simulink model "GOSH1"  (Simulink 8.1)
settings: Solver=ode45  StartTime=0.0  StopTime=10.0  RelTol=1e-3
libraries: simulink x1
settings Model: Creator=Mihail  LastModifiedBy=Mihail
settings DebuggingCC: FcnCallInpInsideContextMsg=EnableAllAsWarning
settings GRTTargetCC: CombineOutputUpdateFcns=on  GRTInterface=off

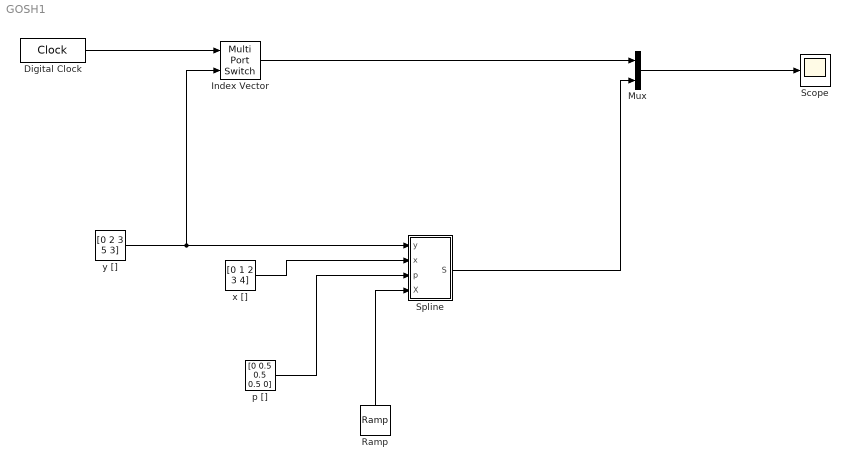
== system GOSH1 ==
  Digital Clock : DigitalClock
  Index Vector : MultiPortSwitch  DataPortOrder=Zero-based contiguous  Inputs=1  zeroidx=on
  Mux : Mux  Inputs=2
  Ramp : simulink/Sources/Ramp  slope=1  start=0  X0=0
  Scope : Scope
      settings: TimeRange=0.06668296375670701  YMin=2.961430172622083  YMax=3.275129869258235
  Spline : Subsystem
  p [] : Constant  Value=[0 0.5 0.5 0.5 0]
  x [] : Constant  Value=[0 1 2 3 4]
  y [] : Constant  Value=[0 2 3 5 3]
  wires:
  y []/1 -> Index Vector/2, Spline/1(y)
  Index Vector/1 -> Mux/1
  Digital Clock/1 -> Index Vector/1
  Mux/1 -> Scope/1
  x []/1 -> Spline/2(x)
  Ramp/1 -> Spline/4(X)
  Spline/1(S) -> Mux/2
  p []/1 -> Spline/3(p)

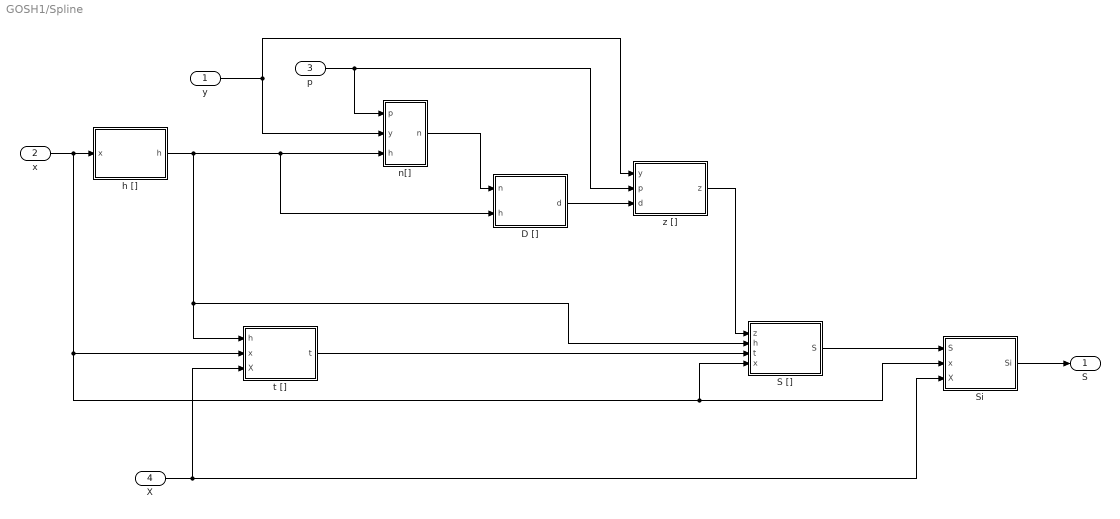
== system GOSH1/Spline ==
  y : Inport
  x : Inport  Port=2
  p : Inport  Port=3
  X : Inport  Port=4
  D [] : MATLAB Function  TreatAsAtomicUnit=on
  S [] : MATLAB Function  TreatAsAtomicUnit=on
  Si : MATLAB Function  TreatAsAtomicUnit=on
  h [] : MATLAB Function  TreatAsAtomicUnit=on
  n[] : Subsystem
  t [] : MATLAB Function  TreatAsAtomicUnit=on
  z [] : MATLAB Function  TreatAsAtomicUnit=on
  S : Outport
  wires:
  Si/1(Si) -> S/1
  S []/1(S) -> Si/1(S)
  y/1 -> n[]/2(y), z []/1(y)
  n[]/1(n) -> D []/1(n)
  X/1 -> Si/3(X), t []/3(X)
  p/1 -> n[]/1(p), z []/2(p)
  x/1 -> Si/2(x), S []/4(x), t []/2(x), h []/1(x)
  z []/1(z) -> S []/1(z)
  t []/1(t) -> S []/3(t)
  D []/1(d) -> z []/3(d)
  h []/1(h) -> t []/1(h), S []/2(h), D []/2(h), n[]/3(h)

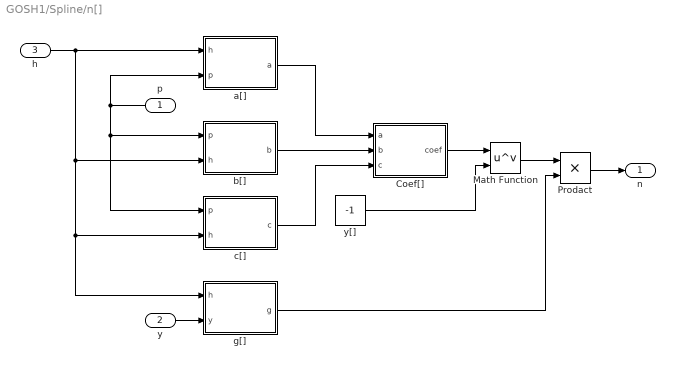
== system GOSH1/Spline/n[] ==
  p : Inport
  y : Inport  Port=2
  h : Inport  Port=3
  Coef[] : MATLAB Function  TreatAsAtomicUnit=on
  Math Function : Math  Operator=pow  SaturateOnIntegerOverflow=on
  Prodact : Product  Inputs=**
  a[] : MATLAB Function  TreatAsAtomicUnit=on
  b[] : MATLAB Function  TreatAsAtomicUnit=on
  c[] : MATLAB Function  TreatAsAtomicUnit=on
  g[] : MATLAB Function  TreatAsAtomicUnit=on
  y[] : Constant  Value=-1
  n : Outport
  wires:
  h/1 -> g[]/1(h), c[]/2(h), b[]/2(h), a[]/1(h)
  y/1 -> g[]/2(y)
  a[]/1(a) -> Coef[]/1(a)
  b[]/1(b) -> Coef[]/2(b)
  c[]/1(c) -> Coef[]/3(c)
  p/1 -> a[]/2(p), b[]/1(p), c[]/1(p)
  y[]/1 -> Math Function/2
  Coef[]/1(coef) -> Math Function/1
  Math Function/1 -> Prodact/1
  g[]/1(g) -> Prodact/2
  Prodact/1 -> n/1

== matlab function Spline/t [] ==
  data: h input double; x input double; t output double; X input double
function t = fcn(h,x,X)
%#codegen
syms X
n=length(h);
for i=1:1:n
    T=[T (X-x(i))/h(i)];
end;
t = T;

== matlab function Spline/h [] ==
  data: x input double; h output double
function h = fcn(x)
%#codegen
n=length(x);
for i=1:1:n-1
    H=[H x(i+1)-x(i)];
end;
h =H;

== matlab function Spline/n[]/a[] ==
  data: h input double; a output double; p input double
function a = fcn(h,p)
%#codegen
n=length(h);
for i=2:1:n
    A=[A (h(i-1)+h(i))/3+p(i-1)/(h(i-1))^2+(1/h(i-1)+1/h(i))^2*p(i)+p(i+1)/(h(i)^2)];
end;
a = [1 A 1];

== matlab function Spline/n[]/b[] ==
  data: p input double; h input double; b output double
function b = fcn(p,h)
%#codegen
n=length(h)-1;
for i=2:1:n
    B=[B h(i)/6-((1/h(i-1)+1/h(i))*p(i)  +  ((1/h(i+1)+1/h(i))*p(i+1)))/h(i)];
end;
b = [1 B 1];

== matlab function Spline/n[]/c[] ==
  data: p input double; h input double; c output double
function c = fcn(p,h)
%#codegen
n=length(h)-2;
for i=2:1:n
   C=[C 1/(h(i)*h(i+1))*p(i+1)];
end;
c = [0 C 0];

== matlab function Spline/n[]/g[] ==
  data: h input double; g output double; y input double
function g = fcn(h,y)
%#codegen
n=length(h);
for i=2:1:n
   G=[G 1/(h(i)*h(i+1))*p(i+1)];
end;
g = [0 G 0];

== matlab function Spline/n[]/Coef[] ==
  data: a input double; b input double; c input double; coef output double
function coef = fcn(a,b,c)
%#codegen
m=length(a);
Coef=eye(m,m);
Coef(1,2)=1;
Coef(2,1)=1;
Coef(2,2)=a(2);
Coef(2,3)=b(2);
Coef(2,4)=c(2);
for i=3:1:m-2
    Coef(i,i-2)=c(i-2);
    Coef(i,i-1)=b(i-1);
    Coef(i,i)=a(i);
    Coef(i,i+1)=b(i);
    Coef(i,i+2)=c(i);
end;
Coef(m-1,m-3)=c(m-3);
Coef(m-1,m-2)=b(m-2);
Coef(m-1,m-1)=a(m-1);
Coef(m-1,m)=b(m-1);

Coef(m,m-1)=1;
coef=Coef;

== matlab function Spline/D [] ==
  data: n input double; h input double; d output double
function d = fcn(n,h)
%#codegen
m=length(n);
D0=1/h(1)*(n(2)-n(0));
Dm=-1/(h(m-1))*(n(m)-n(m-1));
for i=2:1:m-1
    d=(h(i-1)+h(i))/3+p(i-1)/(h(i-1))^2+(1/h(i-1)+1/h(i))^2*p(i)+p(i+1)/(h(i)^2);
end;
d = [D0 D Dm];

== matlab function Spline/z [] ==
  data: y input double; p input double; d input double; z output double
function z = fcn(y,p,d)
%#codegen
for i=1:1:length(y)
    Z=[Z y(i)-p(i)*d(i)];
end;
z =Z;

== matlab function Spline/S [] ==
  data: z input double; h input double; t input double; x input double; S output double
function S = fcn(z,h,t,x)
%#codegen
syms X
n=length(t);
for i=1:1:n
    s=z(i)*(1-t(i))+z(i+1)t(i)
end;
S = T;

== matlab function Spline/Si ==
  data: S input double; x input double; X input double; Si output double
function Si = fcn(S,x,X)
%#codegen
syms X
n=length(x);
p=0;
for i=1:1:n
    if((x(i)>X)&&(p~=0))
        p=i;
    end;
end;
Si = S(p);
